simulink library "halin"  (R2024a)
settings: Solver=VariableStepAuto  StartTime=0.0  StopTime=10.0  RelTol=1e-3
undefined symbols (not defined in the file): KHAL_CAN3BMS1E2E_flg, KHAL_CAN3BMS6E2E_flg, TimeoutOccurred
libraries: FVT_lib x12, simulink x6, hcu_lib x1
(part 2 of 2)

== system halin/HAL_IN/CAN_MCU_R1/EOP_FVT_R_Local1/EOPFVTRActualSpdSta ==
  EOP_FVT_R_ActualSpd_Sta : Inport
  UnitConverter : DataTypeConversion  OutDataTypeStr=uint16  SaturateOnIntegerOverflow=off  RndMeth=Floor
  VHAL_EOPFVTRActualSpdSta_rpm : Outport
  wires:
  UnitConverter/1 -> VHAL_EOPFVTRActualSpdSta_rpm/1
  EOP_FVT_R_ActualSpd_Sta/1 -> UnitConverter/1

== system halin/HAL_IN/CAN_MCU_R1/EOP_FVT_R_Local1/EOPFVTRCSInvalidSta ==
  EOP_FVT_R_CSInvalid_Sta : Inport
  UnitConverter : DataTypeConversion  OutDataTypeStr=uint8  SaturateOnIntegerOverflow=off  RndMeth=Floor
  VHAL_EOPFVTRCSInvalidSta_flg : Outport
  wires:
  UnitConverter/1 -> VHAL_EOPFVTRCSInvalidSta_flg/1
  EOP_FVT_R_CSInvalid_Sta/1 -> UnitConverter/1

== system halin/HAL_IN/CAN_MCU_R1/EOP_FVT_R_Local1/EOPFVTRCanLossSta ==
  EOP_FVT_R_CanLoss_Sta : Inport
  UnitConverter : DataTypeConversion  OutDataTypeStr=uint8  SaturateOnIntegerOverflow=off  RndMeth=Floor
  VHAL_EOPFVTRCanLossSta_flg : Outport
  wires:
  UnitConverter/1 -> VHAL_EOPFVTRCanLossSta_flg/1
  EOP_FVT_R_CanLoss_Sta/1 -> UnitConverter/1

== system halin/HAL_IN/CAN_MCU_R1/EOP_FVT_R_Local1/EOPFVTREnableOffSta ==
  EOP_FVT_R_EnableOff_Sta : Inport
  UnitConverter : DataTypeConversion  OutDataTypeStr=uint8  SaturateOnIntegerOverflow=off  RndMeth=Floor
  VHAL_EOPFVTREnableOffSta_flg : Outport
  wires:
  UnitConverter/1 -> VHAL_EOPFVTREnableOffSta_flg/1
  EOP_FVT_R_EnableOff_Sta/1 -> UnitConverter/1

== system halin/HAL_IN/CAN_MCU_R1/EOP_FVT_R_Local1/EOPFVTRHallSigErrSta ==
  EOP_FVT_R_HallSigErr_Sta : Inport
  UnitConverter : DataTypeConversion  OutDataTypeStr=uint8  SaturateOnIntegerOverflow=off  RndMeth=Floor
  VHAL_EOPFVTRHallSigErrSta_flg : Outport
  wires:
  UnitConverter/1 -> VHAL_EOPFVTRHallSigErrSta_flg/1
  EOP_FVT_R_HallSigErr_Sta/1 -> UnitConverter/1

== system halin/HAL_IN/CAN_MCU_R1/EOP_FVT_R_Local1/EOPFVTRLocal1CSSta ==
  EOP_FVT_R_Local1_CS_Sta : Inport
  UnitConverter : DataTypeConversion  OutDataTypeStr=uint8  SaturateOnIntegerOverflow=off  RndMeth=Floor
  VHAL_EOPFVTRLocal1CSSta_enum : Outport
  wires:
  UnitConverter/1 -> VHAL_EOPFVTRLocal1CSSta_enum/1
  EOP_FVT_R_Local1_CS_Sta/1 -> UnitConverter/1

== system halin/HAL_IN/CAN_MCU_R1/EOP_FVT_R_Local1/EOPFVTRLocal1RCSta ==
  EOP_FVT_R_Local1_RC_Sta : Inport
  UnitConverter : DataTypeConversion  OutDataTypeStr=uint8  SaturateOnIntegerOverflow=off  RndMeth=Floor
  VHAL_EOPFVTRLocal1RCSta_enum : Outport
  wires:
  UnitConverter/1 -> VHAL_EOPFVTRLocal1RCSta_enum/1
  EOP_FVT_R_Local1_RC_Sta/1 -> UnitConverter/1

== system halin/HAL_IN/CAN_MCU_R1/EOP_FVT_R_Local1/EOPFVTROverTempBCKSta ==
  EOP_FVT_R_OverTempBCK_Sta : Inport
  UnitConverter : DataTypeConversion  OutDataTypeStr=uint8  SaturateOnIntegerOverflow=off  RndMeth=Floor
  VHAL_EOPFVTROverTempBCKSta_enum : Outport
  wires:
  UnitConverter/1 -> VHAL_EOPFVTROverTempBCKSta_enum/1
  EOP_FVT_R_OverTempBCK_Sta/1 -> UnitConverter/1

== system halin/HAL_IN/CAN_MCU_R1/EOP_FVT_R_Local1/EOPFVTROverTempSta ==
  EOP_FVT_R_OverTemp_Sta : Inport
  UnitConverter : DataTypeConversion  OutDataTypeStr=uint8  SaturateOnIntegerOverflow=off  RndMeth=Floor
  VHAL_EOPFVTROverTempSta_flg : Outport
  wires:
  UnitConverter/1 -> VHAL_EOPFVTROverTempSta_flg/1
  EOP_FVT_R_OverTemp_Sta/1 -> UnitConverter/1

== system halin/HAL_IN/CAN_MCU_R1/EOP_FVT_R_Local1/EOPFVTROverVolSta ==
  EOP_FVT_R_OverVol_Sta : Inport
  UnitConverter : DataTypeConversion  OutDataTypeStr=uint8  SaturateOnIntegerOverflow=off  RndMeth=Floor
  VHAL_EOPFVTROverVolSta_enum : Outport
  wires:
  UnitConverter/1 -> VHAL_EOPFVTROverVolSta_enum/1
  EOP_FVT_R_OverVol_Sta/1 -> UnitConverter/1

== system halin/HAL_IN/CAN_MCU_R1/EOP_FVT_R_Local1/EOPFVTRPumpReadySta ==
  EOP_FVT_R_PumpReady_Sta : Inport
  UnitConverter : DataTypeConversion  OutDataTypeStr=uint8  SaturateOnIntegerOverflow=off  RndMeth=Floor
  VHAL_EOPFVTRPumpReadySta_flg : Outport
  wires:
  UnitConverter/1 -> VHAL_EOPFVTRPumpReadySta_flg/1
  EOP_FVT_R_PumpReady_Sta/1 -> UnitConverter/1

== system halin/HAL_IN/CAN_MCU_R1/EOP_FVT_R_Local1/EOPFVTRRCInvalidSta ==
  EOP_FVT_R_RCInvalid_Sta : Inport
  UnitConverter : DataTypeConversion  OutDataTypeStr=uint8  SaturateOnIntegerOverflow=off  RndMeth=Floor
  VHAL_EOPFVTRRCInvalidSta_flg : Outport
  wires:
  UnitConverter/1 -> VHAL_EOPFVTRRCInvalidSta_flg/1
  EOP_FVT_R_RCInvalid_Sta/1 -> UnitConverter/1

== system halin/HAL_IN/CAN_MCU_R1/EOP_FVT_R_Local1/EOPFVTRRunStatusSta ==
  EOP_FVT_R_RunStatus_Sta : Inport
  UnitConverter : DataTypeConversion  OutDataTypeStr=uint8  SaturateOnIntegerOverflow=off  RndMeth=Floor
  VHAL_EOPFVTRRunStatusSta_enum : Outport
  wires:
  UnitConverter/1 -> VHAL_EOPFVTRRunStatusSta_enum/1
  EOP_FVT_R_RunStatus_Sta/1 -> UnitConverter/1

== system halin/HAL_IN/CAN_MCU_R1/EOP_FVT_R_Local1/EOPFVTRStartFailureSta ==
  EOP_FVT_R_StartFailure_Sta : Inport
  UnitConverter : DataTypeConversion  OutDataTypeStr=uint8  SaturateOnIntegerOverflow=off  RndMeth=Floor
  VHAL_EOPFVTRStartFailureSta_flg : Outport
  wires:
  UnitConverter/1 -> VHAL_EOPFVTRStartFailureSta_flg/1
  EOP_FVT_R_StartFailure_Sta/1 -> UnitConverter/1

== system halin/HAL_IN/CAN_MCU_R1/EOP_FVT_R_Local1/EOPFVTRUnderVolSta ==
  EOP_FVT_R_UnderVol_Sta : Inport
  UnitConverter : DataTypeConversion  OutDataTypeStr=uint8  SaturateOnIntegerOverflow=off  RndMeth=Floor
  VHAL_EOPFVTRUnderVolSta_enum : Outport
  wires:
  UnitConverter/1 -> VHAL_EOPFVTRUnderVolSta_enum/1
  EOP_FVT_R_UnderVol_Sta/1 -> UnitConverter/1
